simulink model "simulinkRLC"  (R2023a)
settings: Solver=VariableStepAuto  StartTime=0.0  StopTime=.01  RelTol=1e-3
values from neighbouring files (symbols this model uses):
  C = 0.000010    (= 1e-05)    [CDCD.m]    (also in CDCD_Parametros.m; C_RLC.m = 1e-07; Grafico_circuito_RLC.m = 1e-07; Practica2.m = [c1 -m2*l2*x(4)*sin(x(2)-x(1));l1*x(3)*sin(x(2)-x(1)) 0])
  frec = 500    [RLC_Parameters.m]
  L = 0.002    [CDCD.m]    (also in CDCD_Parametros.m; C_RLC.m = 0.006; MotorDC.m = 0.023; Parametros_Motor.m = 0.023)
  R = 10    [CDCD.m]    (also in CDCD_Parametros.m; C_RLC.m = 100; MotorDC.m = 2; Parametros_Motor.m = 2)
libraries: ee_lib x3, fl_lib x3, nesl_utility x3
settings Model: Creator=ferch  LastModifiedBy=mluser
settings OptimizationCC: ReuseModelBlockBuffer=off

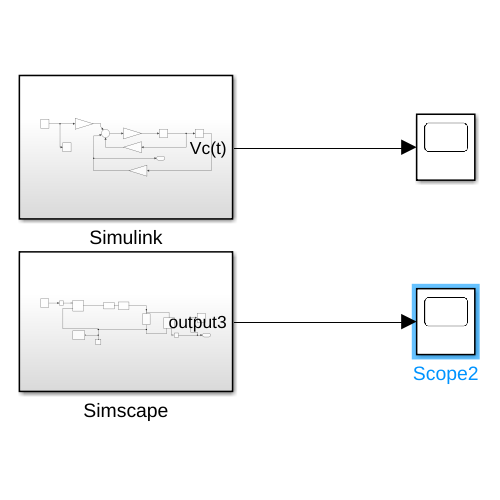
[thumbnail: Simulink's stored preview of the top-level diagram]
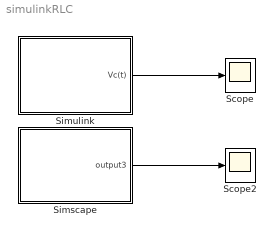
== system simulinkRLC ==
  Scope : Scope
  Scope2 : Scope
  Simscape : Subsystem
  Simulink : Subsystem
  wires:
  Simulink/1(Vc(t)) -> Scope/1
  Simscape/1(output3) -> Scope2/1

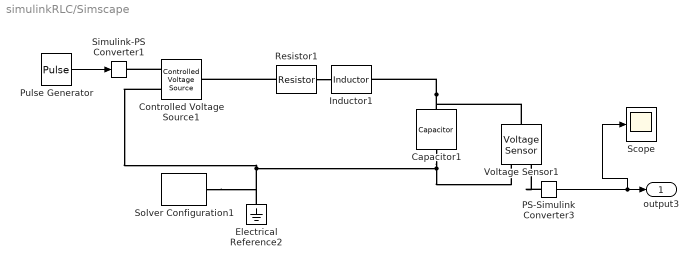
== system simulinkRLC/Simscape ==
  Capacitor1 : ee_lib/Passive/Capacitor  cap_option=0  c=.1 uF  Cvec=[1e-05, 1e-06] F  Vvec=[0, 10] V  CV_table_symmetry=1  f_vec=[1, 10] kHz  DFext_vec=[.8, 1.2]  enable_C_tol=0  averaging_period=0 s  C_tol=5  tol_distribution=1  nSigma=4  r=1e-6 Ohm  g=0 1/Ohm  enable_operating_limits=0  enable_faults=ee.enum.enable.no  fault_action=simscape.enum.assert.action.none  Cscale_faulted=100  R_faulted=1e-3 Ohm  G_faulted=0 1/Ohm  tau_fault=1e-3 s  fault_trigger=ee.enum.faults.faultTrigger.temporal  t_fault=1 s  max_permissible_voltage_range=[-100, 100] V  t_fail_on_voltage=1 s  operating_limit_action=2  max_working_voltage_range=[-25, 25] V  power_rating=1 W  i_specify=off  i_priority=None  i=0 A  i_nominal_specify=off  i_nominal_unit=A  i_nominal_value=1  v_specify=off  v_priority=None  v=0 V  v_nominal_specify=off  v_nominal_unit=V  v_nominal_value=1  vc_specify=off  vc_priority=High  vc=0 V  vc_nominal_specify=off  vc_nominal_unit=V  vc_nominal_value=1
  Controlled Voltage Source1 : fl_lib/Electrical/Electrical Sources/Controlled Voltage Source
  Electrical Reference2 : fl_lib/Electrical/Electrical Elements/Electrical Reference
  Inductor1 : ee_lib/Passive/Inductor  l=4.13 mH  enable_L_tol=0  L_tol=20  tol_distribution=1  nSigma=4  r=0 Ohm  g=1e-9 1/Ohm  enable_operating_limits=0  operating_limit_action=2  max_working_current=1 A  power_rating=1 W  enable_faults=ee.enum.enable.no  fault_action=simscape.enum.assert.action.none  lambdaPercent=50  k_faulted=0.9999  turnsShort=0  openCct=0  groundShort=0  groundShortG=0 1/Ohm  tau_fault=1e-3 s  fault_trigger=ee.enum.faults.faultTrigger.temporal  t_fault=1 s  max_permissible_voltage=100 V  n_fail_on_voltage=1  max_permissible_current=1 A  t_fail_on_current=1 s  i_L_specify=off  i_L_priority=High  i_L=0 A  i_L_nominal_specify=off  i_L_nominal_unit=A  i_L_nominal_value=1
  PS-Simulink Converter3 : nesl_utility/PS-Simulink Converter  PhysicalDomain=network_engine_domain  SubClassName=ps_output  LeftPortType=input  RightPortType=output  PseudoPeriodic=off  Frequencies=[]  VectorFormat=inherit  Unit=inherit  AffineConversion=off
  Pulse Generator : DiscretePulseGenerator  PulseType=Time based  Amplitude=12  Period=0.002  PulseWidth=50
  Resistor1 : ee_lib/Passive/Resistor  R=122 Ohm  enable_R_tol=0  R_tol=5  tol_distribution=1  nSigma=4  enable_operating_limits=0  operating_limit_action=2  power_rating=1 W  max_working_voltage=100 V  enable_faults=ee.enum.enable.no  fault_action=simscape.enum.assert.action.none  R_faulted=inf Ohm  fault_trigger=ee.enum.faults.faultTrigger.temporal  t_fault=1 s  max_permissible_current=1 A  t_fail_on_current=1 s  noise_mode=0  Tdevice=25 degC  sample_time=1e-3 s  repeatability=1  user_seed=0  auto_seed=3890346746  power_derating_T1=70 degC  power_derating_T2=155 degC  operating_temperature_range_vec=[-50, 150] degC  alpha=3.93e-3 1/K  Tmeas=25 degC  thermal_mass=100 J/K  temperature_specify=off  temperature_priority=High  temperature=298.15 K  temperature_nominal_specify=off  temperature_nominal_unit=K  temperature_nominal_value=1
  Scope : Scope
  Simulink-PS Converter1 : nesl_utility/Simulink-PS Converter  PhysicalDomain=network_engine_domain  SubClassName=ps_input  LeftPortType=input  RightPortType=output  PseudoPeriodic=off  Frequencies=[]  NoiseDistribution=none  NoiseParameters=[]  Unit=1  AffineConversion=off  FilteringAndDerivatives=provide  SimscapeFilterOrder=1  InputFilterTimeConstant=0.001  UdotUserProvided=0
  Solver Configuration1 : nesl_utility/Solver Configuration  PhysicalDomain=network_engine_domain  SubClassName=solver  LeftPortType=input  RightPortType=generic  Tones=[]  Harmonics=[]  SimulateNoise=off  Profile=off  UseLocalSampling=off  EnableSwitchedLinearOptims=on  FrequencyDomain=off  UseCCode=off  RelTol=0.001  AbsTol=0.001  MinStep=1e-09  ToWorkspace=off  RevertToSquareIcSolve=off  NumHomotopyIterations=100  PhasorMode=off  PhasorModeNumHarmonics=1  ConsistencySolver=NEWTON_XTOL_AFTER_FTOL  IndexReductionMethod=DerivativeReplacement  DoDC=off  ResidualTolerance=1e-09  ConsistencyTolSource=GLOBAL  ConsistencyAbsTol=0.001  ConsistencyRelTol=0.001  ConsistencyTolFactor=0.001  UseLocalSolver=off  LocalSolverChoice=NE_BACKWARD_EULER_ADVANCER  ResolveIndetEquations=on  FunctionEvalNumThread=1  LocalSolverSampleTime=0.001  DoFixedCost=off  MaxNonlinIter=3  MaxModeIter=2  ComputeImpulses=off  ImpulseIterations=2  LinearAlgebra=auto  LinearAlgebraNumThread=0  EquationFormulation=NE_TIME_EF  DelaysMemoryBudget=1024  AutomaticFiltering=on  FilteringTimeConstant=0.001  PartitionStorageMethod=AS_NEEDED  PartitionMemoryBudget=1024  PartitionMethod=ROBUST
  Voltage Sensor1 : fl_lib/Electrical/Electrical Sensors/Voltage Sensor
  output3 : Outport
  wires:
  Pulse Generator/1 -> Simulink-PS Converter1/1
  PS-Simulink Converter3/1 -> Scope/1, output3/1
  connections:
  Voltage Sensor1/LConn1 -- Capacitor1/LConn1 -- Inductor1/RConn1
  Controlled Voltage Source1/RConn1 -- Simulink-PS Converter1/RConn1
  PS-Simulink Converter3/LConn1 -- Voltage Sensor1/RConn1
  Resistor1/RConn1 -- Controlled Voltage Source1/LConn1
  Resistor1/LConn1 -- Inductor1/LConn1
  Capacitor1/RConn1 -- Voltage Sensor1/RConn2 -- Solver Configuration1/RConn1 -- Electrical Reference2/LConn1 -- Controlled Voltage Source1/RConn2

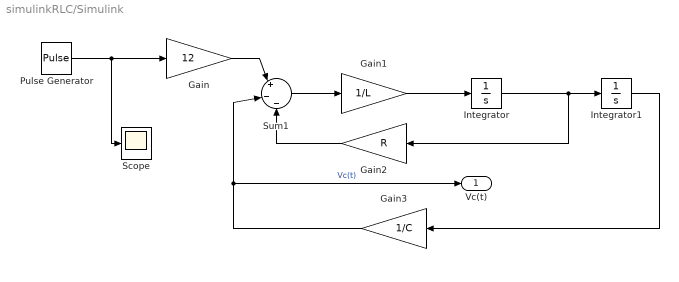
== system simulinkRLC/Simulink ==
  Gain : Gain  Gain=12
  Gain1 : Gain  Gain=1/L
  Gain2 : Gain  Gain=R
  Gain3 : Gain  Gain=1/C
  Integrator : Integrator
  Integrator1 : Integrator
  Pulse Generator : DiscretePulseGenerator  PulseType=Time based  Period=1/frec  PulseWidth=50
  Scope : Scope
  Sum1 : Sum  Inputs=|+|-|-
  Vc(t) : Outport
  wires:
  Integrator1/1 -> Gain3/1
  Gain/1 -> Sum1/1
  Gain3/1 -> Vc(t)/1, Sum1/2  "Vc(t)"
  Integrator/1 -> Gain2/1, Integrator1/1
  Gain2/1 -> Sum1/3
  Gain1/1 -> Integrator/1
  Pulse Generator/1 -> Scope/1, Gain/1
  Sum1/1 -> Gain1/1
